simulink model "BeagleBone_Testing"  (R2024a)
settings: Solver=VariableStepAuto  StartTime=0.0  StopTime=10.0  RelTol=1e-3
undefined symbols (not defined in the file): Discrete, R, Time
libraries: bbblueActuatorLib x4, ctrlSharedLib x1, bbblueSensorLib x1
settings Model: Creator=eduar  LastModifiedBy=eduar

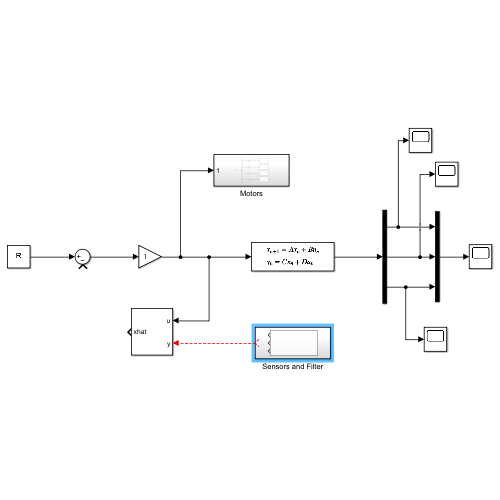
[thumbnail: Simulink's stored preview of the top-level diagram]
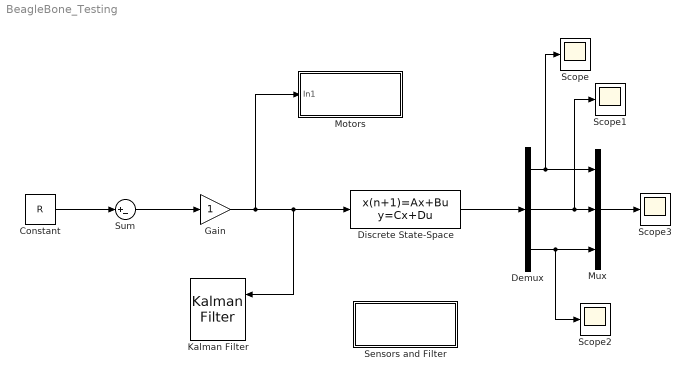
== system BeagleBone_Testing ==
  Constant : Constant  Value=R
  Demux : Demux  Outputs=3
  Discrete State-Space : DiscreteStateSpace  SampleTime=-1
  Gain : Gain
  Kalman Filter : ctrlSharedLib/Kalman Filter  TimeDomain=Discrete-Time  UseCurrentEstimator=on  ModelSource=LTI State-Space Variable  ModelSourceVariable=ss(0.95,1,1,0,1)  A=0.95  B=1  C=1  D=0  NumberOfStates=1  NumberOfInputs=1  NumberOfOutputs=1  InitialEstimateSource=Dialog  X0=0  P0=10  UseK=off  UseGH=off  NumberOfProcessNoiseInputs=1  G=1  TimeInvariantG=on  H=0  TimeInvariantH=on  Q=0.05  TimeInvariantQ=on  R=1  TimeInvariantR=on  N=0  TimeInvariantN=on  AddInputPort=on  AddEnablePort=off  OutputEstimatedY=off  OutputP=off  Ts=-1
  Motors : Subsystem
  Mux : Mux  Inputs=3
  Scope{,1..3} (4 alike) : Scope
  Sensors and Filter : Subsystem
  Sum : Sum  Inputs=|+-
  wires:
  Constant/1 -> Sum/1
  Sum/1 -> Gain/1
  Gain/1 -> Motors/1(In1), Kalman Filter/1, Discrete State-Space/1
  Demux/1 -> Mux/1, Scope/1
  Discrete State-Space/1 -> Demux/1
  Demux/2 -> Scope1/1, Mux/2
  Demux/3 -> Scope2/1, Mux/3
  Mux/1 -> Scope3/1
  ? -> Kalman Filter/2

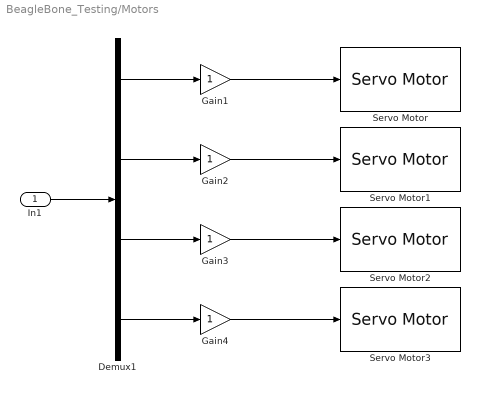
== system BeagleBone_Testing/Motors ==
  In1 : Inport
  Demux1 : Demux
  Gain{1..4} (4 alike) : Gain
  Servo Motor : bbblueActuatorLib/Servo Motor  channel=1  SimulateUsing=Code generation
  Servo Motor1 : bbblueActuatorLib/Servo Motor  channel=2  SimulateUsing=Code generation
  Servo Motor2 : bbblueActuatorLib/Servo Motor  channel=3  SimulateUsing=Code generation
  Servo Motor3 : bbblueActuatorLib/Servo Motor  channel=4  SimulateUsing=Code generation
  wires:
  Gain2/1 -> Servo Motor1/1
  Gain3/1 -> Servo Motor2/1
  Demux1/1 -> Gain1/1
  Gain4/1 -> Servo Motor3/1
  Gain1/1 -> Servo Motor/1
  Demux1/4 -> Gain4/1
  Demux1/2 -> Gain2/1
  Demux1/3 -> Gain3/1
  In1/1 -> Demux1/1

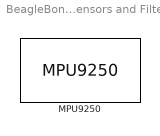
== system BeagleBone_Testing/Sensors and Filter ==
  MPU9250 : bbblueSensorLib/MPU9250  OperationMode=DMP  Accel=on  AngularRate=on  Ak8963Field=on  EulerAngles=off  Quat=off  AccelRange=2G  Acceldlpf=1  GyroRange=250 dps  Gyrodlpf=1  DmpOdr=200 Hz  SampleTime=0.1
